simulink model "legocar"  (R2015b)
settings: Solver=VariableStepAuto  StartTime=0.0  StopTime=0.2  RelTol=1e-5
values from neighbouring files (symbols this model uses):
  alpha = u_mpc(2)    [controller.m]    (also in controller_lqr.m; controller_lqr2.m; controller_mpc_Tunner.m)
  v = u_mpc(1)    [controller.m]    (also in controller_lqr.m; sim_veh_MPC.m = v_state.Data(h); sim_veh_MPC_smooth.m = v_state.Data(h))
  x_car0 = x_car    (= 0)    [sim_veh_MPC.m]    (also in sim_veh_MPC_smooth.m)
  y_car0 = y_car    (= 0)    [sim_veh_MPC.m]    (also in sim_veh_MPC_smooth.m)
undefined symbols (not defined in the file or in its folder): theta0
settings Model: Creator=Jesse  LastModifiedBy=Jesse

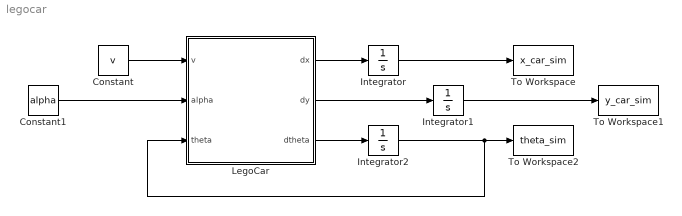
== system legocar ==
  Constant : Constant  Value=v
  Constant1 : Constant  Value=alpha
  Integrator : Integrator  InitialCondition=x_car0
  Integrator1 : Integrator  InitialCondition=y_car0
  Integrator2 : Integrator  InitialCondition=theta0
  LegoCar : MATLAB Function  TreatAsAtomicUnit=on
  To Workspace : ToWorkspace  VariableName=x_car_sim  SaveFormat=Timeseries  SampleTime=-1
  To Workspace1 : ToWorkspace  VariableName=y_car_sim  SaveFormat=Timeseries  SampleTime=-1
  To Workspace2 : ToWorkspace  VariableName=theta_sim  SaveFormat=Timeseries  SampleTime=-1
  wires:
  LegoCar/3(dtheta) -> Integrator2/1
  Integrator2/1 -> To Workspace2/1, LegoCar/3(theta)
  LegoCar/2(dy) -> Integrator1/1
  LegoCar/1(dx) -> Integrator/1
  Constant/1 -> LegoCar/1(v)
  Constant1/1 -> LegoCar/2(alpha)
  Integrator/1 -> To Workspace/1
  Integrator1/1 -> To Workspace1/1

== matlab function legocar/LegoCar ==
  data: v input; dx output; alpha input; theta input; dy output; dtheta output
function [dx,dy,dtheta] = fcn(v,alpha,theta)
l = 11.1;
dx = v*cos(theta);
dy = v*sin(theta);
dtheta = v/l*tan(-alpha);
